simulink model "V5_SUB_DC_DC_Wandler_Validierung"  (R2022b)
settings: Solver=VariableStepAuto  StartTime=0.0  StopTime=10.0  RelTol=1e-3
settings Model: Creator=janbe  LastModifiedBy=janbe

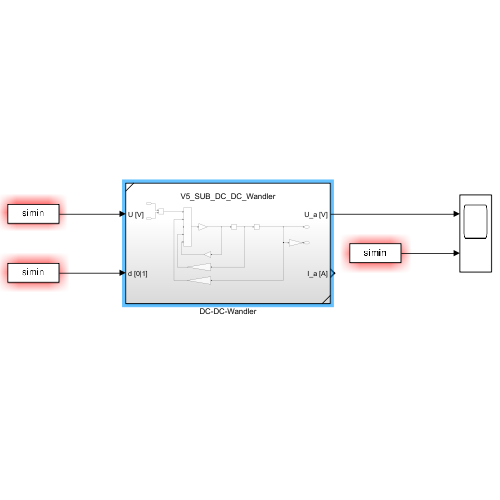
[thumbnail: Simulink's stored preview of the top-level diagram]
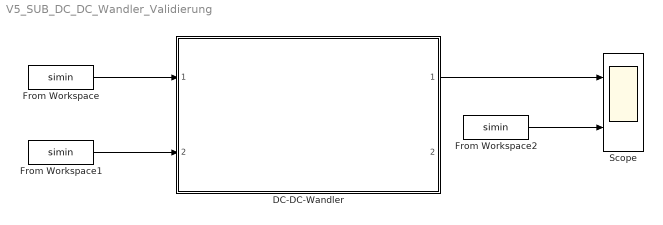
== system V5_SUB_DC_DC_Wandler_Validierung ==
  DC-DC-Wandler : Subsystem  ReferencedSubsystem=V5_SUB_DC_DC_Wandler
  From Workspace : FromWorkspace  VariableName=simin
  From Workspace1 : FromWorkspace  VariableName=simin
  From Workspace2 : FromWorkspace  VariableName=simin
  Scope : Scope  NumInputPorts=2
  wires:
  From Workspace/1 -> DC-DC-Wandler/1
  From Workspace1/1 -> DC-DC-Wandler/2
  DC-DC-Wandler/1 -> Scope/1
  From Workspace2/1 -> Scope/2
